simulink model "controller_6dof_container"  (R2025b)
settings: Solver=ode1  StartTime=0.0  StopTime=20  FixedStep=0.005  RelTol=1e-3
InitFcn:
  | params
settings Model: Creator=schwmaxi  LastModifiedBy=schwmaxi
settings DataIOCC: ExternalInput=input_data  SaveOutput=off  SaveTime=off
settings OptimizationCC: UseDivisionForNetSlopeComputation=on  GainParamInheritBuiltInType=on  UseFloatMulNetSlope=on  EnhancedBackFolding=on  BooleansAsBitfields=on  PassReuseOutputArgsAs=Individual arguments  StateBitsets=on  DataBitsets=on  ZeroExternalMemoryAtStartup=off  ZeroInternalMemoryAtStartup=off  NoFixptDivByZeroProtection=on  EfficientFloat2IntCast=on  LifeSpan=1  OptimizeBlockOrder=speed  DifferentSizesBufferReuse=on  EfficientTunableParamExpr=on
settings DebuggingCC: ParameterTunabilityLossMsg=error
settings HardwareCC: ProdBitPerPointer=32.0  ProdBitPerSizeT=32.0  ProdBitPerPtrDiffT=32.0  ProdWordSize=32.0  ProdLongLongMode=on  ProdHWDeviceType=Custom Processor->Custom Processor
settings SFSimCC: MATLABDynamicMemAlloc=off  SimTargetLang=C++  SimDLTargetLibrary=mkl-dnn
settings RTWCC: SystemTargetFile=ert.tlc  GenCodeOnly=on  TemplateMakefile=ert_default_tmf  TargetLang=C++  Description=Embedded Coder
settings CodeAppCC: ForceParamTrailComments=on  IgnoreCustomStorageClasses=off  OperatorAnnotations=on  SimulinkDataObjDesc=on  SFDataObjDesc=on  CustomSymbolStrGlobalVar=rt$N$M  CustomSymbolStrType=$N$M  CustomSymbolStrFcn=$N$M$F  CustomSymbolStrMacro=$N$M  InsertBlockDesc=on
settings ERTTargetCC: InlinedParameterPlacement=Hierarchical  RootIOFormat=Structure reference  ERTCustomFileTemplate=example_file_process.tlc  ERTFilePackagingFormat=CompactWithDataFile  TargetLangStandard=C++11 (ISO)  GenerateSampleERTMain=on  IncludeMdlTerminateFcn=off  CombineSignalStateStructs=on  CodeInterfacePackaging=C++ class  SubcomponentCodeInterfacePackaging=C++ class  SupportNonFinite=off  SupportComplex=off  SupportContinuousTime=on  SupportNonInlinedSFcns=on  SupportVariableSizeSignals=on

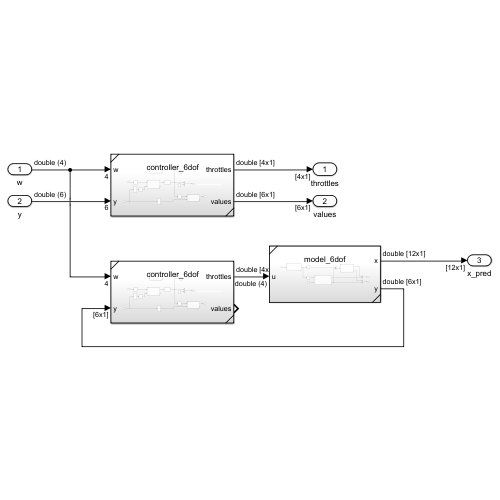
[thumbnail: Simulink's stored preview of the top-level diagram]
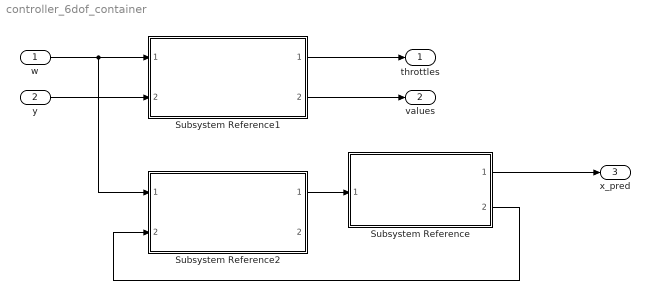
== system controller_6dof_container ==
  w : Inport
  y : Inport  Port=2
  Subsystem Reference : Subsystem  ReferencedSubsystem=model_6dof
  Subsystem Reference1 : Subsystem  ReferencedSubsystem=controller_6dof
  Subsystem Reference2 : Subsystem  ReferencedSubsystem=controller_6dof
  throttles : Outport
  values : Outport  Port=2
  x_pred : Outport  Port=3
  wires:
  Subsystem Reference2/1 -> Subsystem Reference/1
  Subsystem Reference/1 -> x_pred/1
  w/1 -> Subsystem Reference1/1, Subsystem Reference2/1
  y/1 -> Subsystem Reference1/2
  Subsystem Reference1/1 -> throttles/1
  Subsystem Reference/2 -> Subsystem Reference2/2
  Subsystem Reference1/2 -> values/1
